simulink model "lb331_sdruFreqCalibTx"  (R2018b)
settings: Solver=VariableStepAuto  StartTime=0.0  StopTime=inf  RelTol=1e-3
PreLoadFcn:
  | Fs = 200e3; % Частота дискретизации, выборок в с
  | 
  | % Инициализации параметров синусоиды
  | TxSine.Frequency           = 100;
  | TxSine.Amplitude            = 1;
  | TxSine.SamplesPerFrame = 2048;
  | 
  | % Инициализация параметров передачи USRP
  | txradio.MasterClockRate  =  20e6;   % тактовая частота, Гц
  | txradio.CenterFrequency  =  450e6; % центральная частота
  | txradio.Gain                   =  40;       % усиление, дБ
  | % Коэффициент интерполяции
  | txradio.InterpolationFactor = txradio.MasterClockRate/Fs;
libraries: commsdrhw_v2 x1, dspsrcs4 x1
settings Model: Creator=Григорий Фокин  LastModifiedBy=Григорий Фокин
settings SFSimCC: SimUseLocalCustomCode=off
settings RTWCC: RTWUseLocalCustomCode=off
settings CodeAppCC: StateflowObjectComments=on

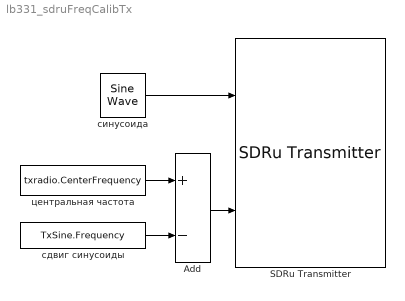
== system lb331_sdruFreqCalibTx ==
  Add : Sum  Inputs=+-
  SDRu Transmitter : commsdrhw_v2/SDRu Transmitter  rxtx=tx  initializeIPAddress=0  devMap=0  USRP2_IP=192.168.10.2  USRP_IP_X300=192.168.10.2  USRP_IP_X310=192.168.10.2  USRP_serialNumB200=No devices found  USRP_serialNumB210=F4E642  platform=B210  prevPlatform=B210  lastIPAddressPopup=192.168.10.2  USRP_ID=F4E642  LastIPAddress=192.168.10.2  ChannelMapping=1  centerFrequencySrc=Input port  centerFrequency=2.45e9  loOffsetSrc=Dialog  loOffset=0  gainSrc=Dialog  gain=txradio.Gain  PPSSource=Internal  clockSource=Internal  masterClkRateParam=20000000  masterClkRateB200=32e6  masterClkRateB210=txradio.MasterClockRate  masterClkRateX300=200e6  masterClkRateX310=200e6  decimInterpSrc=Dialog  decimInterp=txradio.InterpolationFactor  USRP2_IP_NUM=[70 52 69 54 52 50]  frameLength=362  TransportDataType=int16  outputDatatype=Same as transport data type  overrunUnderrunPort=off  sampleTime=1  dboardInfo=|  HOST_DATA_PORT=30000  HOST_CONTROL_PORT=30001  USRP2_DATA_PORT=32769  USRP2_CONTROL_PORT=32768  bufferMode=Continuous streaming  EnableBurstMode=off  NumFramesInBurst=100
      | dbid: 0
      |           dbName: 'no db found'
      |          freqMin: 0
      |          freqMax: 0
      |          gainMin: 0
      |          gainMax: 0
      |     gainStepSize: 0
      settings: SourceProductName=Communications System Toolbox Support Package for USRP(R) Radio  SourceProductBaseCode=USRP
  сдвиг синусоиды : Constant  Value=TxSine.Frequency
  синусоида : dspsrcs4/Sine Wave  Amplitude=TxSine.Amplitude  Frequency=TxSine.Frequency  Phase=0  SampleMode=Discrete  OutComplex=Complex  CompMethod=Trigonometric fcn  TableSize=Speed  SampleTime=1/Fs  SamplesPerFrame=TxSine.SamplesPerFrame  ResetState=Restart at time zero  OutputFrames=off  dataType=double  wordLen=16  udDataType=sfix(16)  fracBitsMode=Best precision  numFracBits=15  OutDataTypeStr=double  LastOutDataTypeStr=double
  центральная частота : Constant  Value=txradio.CenterFrequency
  wires:
  Add/1 -> SDRu Transmitter/2
  центральная частота/1 -> Add/1
  сдвиг синусоиды/1 -> Add/2
  синусоида/1 -> SDRu Transmitter/1
